simulink model "mavsim_chap10"  (R2018b)
settings: Solver=ode15s  StartTime=0.0  StopTime=400  RelTol=1e-3  EnableMultiTasking=on
InitFcn:
  | clearvars
  | path(pathdef)
  | addpath('../chap2_animation')
  | addpath('../parameters/')
  | aerosonde_parameters
  | simulation_parameters
  | wind_parameters
  | sensor_parameters
  | ekf_parameters
  | addpath('../chap3_kinematics')
  | addpath('../chap4_forces')
  | addpath('../chap5_linear')
  | addpath('../chap6_autopilot')
  | compute_autopilot_gains
  | addpath('../chap7_sensors')
  | addpath('../chap8_estimation')
  | addpath('../chap10_follower')
undefined symbols (not defined in the file or in its folder): AP, autopilot, drawPathError, EKF, estimate_states, forces_moments, MAV, path_follow, path_manager_chap10, SENSOR, SIM, true_states, WIND
libraries: simulink x3
settings Model: Creator=beard  LastModifiedBy=Brandon
settings DataIOCC: LimitDataPoints=on  SaveFormat=Array  SignalLoggingSaveFormat=ModelDataLogs
settings OptimizationCC: ExpressionDepthLimit=2147483647  InitFltsAndDblsToZero=on  LifeSpan=inf
settings DebuggingCC: UnderspecifiedInitializationDetection=Classic  MergeDetectMultiDrivingBlocksExec=none  SolverPrmCheckMsg=warning  FcnCallInpInsideContextMsg=warning  AllowSymbolicDim=off  StateNameClashWarn=warning  SFUnexpectedBacktrackingDiag=warning  SFNoUnconditionalDefaultTransitionDiag=warning  SFExecutionAtInitializationDiag=none
settings HardwareCC: ProdBitPerPointer=32  ProdBitPerSizeT=32  ProdBitPerPtrDiffT=32  ProdLargestAtomicFloat=None  ProdIntDivRoundTo=Undefined  ProdEndianess=Unspecified  ProdWordSize=32  ProdHWDeviceType=32-bit Generic
settings ModelReferenceCC: PropagateSignalLabelsOutOfModel=off
settings SFSimCC: SimUseLocalCustomCode=off  SimParseCustomCode=off
settings RTWCC: RTWUseLocalCustomCode=off
settings CodeAppCC: StateflowObjectComments=on
settings GRTTargetCC: TargetLangStandard=C89/C90 (ANSI)  GeneratePreprocessorConditionals=Disable all  CombineOutputUpdateFcns=off  GRTInterface=on
settings ConfigComp: CovMetricSettings=dw  CovHtmlReporting=on  CovSaveCumulativeToWorkspaceVar=on  CovSaveSingleToWorkspaceVar=on  CovExternalEMLEnable=off  CovSFcnEnable=off

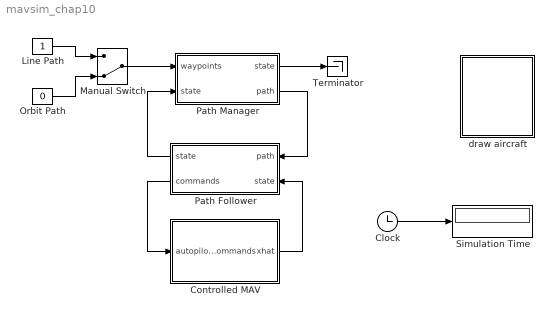
== system mavsim_chap10 ==
  Clock : Clock
  Controlled MAV : Subsystem
      mask Display: image(imread('batcam.png'))
  Line Path : Constant
      settings: AttributesFormatString=%<Name>
  Manual Switch : ManualSwitch  CurrentSetting=0
  Orbit Path : Constant  Value=0
      settings: AttributesFormatString=%<Name>
  Path Follower : Subsystem
  Path Manager : Subsystem
  Simulation Time : Display
  Terminator : Terminator
  draw aircraft : Subsystem
      mask Display: image(imread('tv.jpg'))
  wires:
  Clock/1 -> Simulation Time/1
  Path Manager/2(path) -> Path Follower/1(path)
  Path Follower/2(commands) -> Controlled MAV/1(autopilot commands)
  Controlled MAV/1(xhat) -> Path Follower/2(state)
  Path Follower/1("state ") -> Path Manager/2(state)
  Path Manager/1("state ") -> Terminator/1
  Line Path/1 -> Manual Switch/1
  Orbit Path/1 -> Manual Switch/2
  Manual Switch/1 -> Path Manager/1(waypoints)

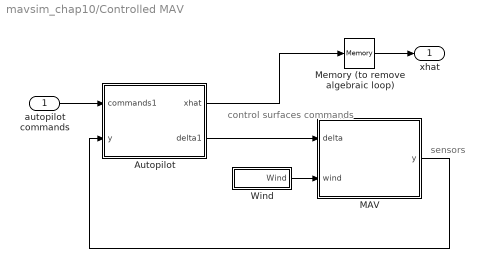
== system mavsim_chap10/Controlled MAV ==
  note: sensors
  note: control surfaces
      | commands
  autopilot commands : Inport
  Autopilot : Subsystem
      mask Display: image(imread('kestrel.jpg'))
  MAV : Subsystem
      mask Display: image(imread('batcam.png'))
  Memory (to remove algebraic loop) : Memory
  Wind : Subsystem
  xhat : Outport
  wires:
  Wind/1(Wind) -> MAV/2(wind)
  MAV/1(y) -> Autopilot/2(y)
  autopilot commands/1 -> Autopilot/1(commands1)
  Memory (to remove algebraic loop)/1 -> xhat/1
  Autopilot/2(delta1) -> MAV/1(delta)
  Autopilot/1(xhat) -> Memory (to remove algebraic loop)/1

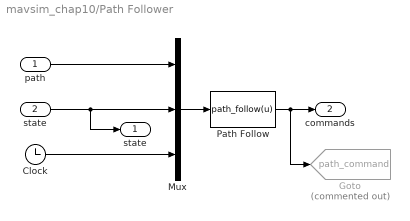
== system mavsim_chap10/Path Follower ==
  path : Inport
  state : Inport  Port=2
  Clock : Clock
  Goto : Goto  Commented=on  GotoTag=path_command  TagVisibility=global
  Mux : Mux  Inputs=3
  Path Follow : MATLABFcn  MATLABFcn=path_follow(u)  OutputDimensions=4  SampleTime=SIM.ts_control
  "state " : Outport
  commands : Outport  Port=2
  wires:
  Path Follow/1 -> commands/1, Goto/1
  Mux/1 -> Path Follow/1
  path/1 -> Mux/1
  Clock/1 -> Mux/3
  state/1 -> Mux/2, "state "/1

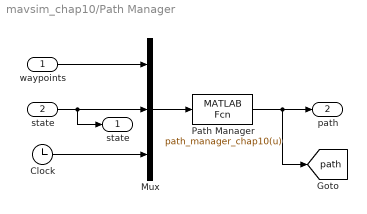
== system mavsim_chap10/Path Manager ==
  waypoints : Inport
  state : Inport  Port=2
  Clock : Clock
  Mux : Mux  Inputs=3
  Path Manager : MATLABFcn  MATLABFcn=path_manager_chap10(u)  OutputDimensions=13  SampleTime=SIM.ts_control
  "state " : Outport
  path : Outport  Port=2
  tag scope: path=global
  wires:
  Path Manager/1 -> path/1, [path]
  Mux/1 -> Path Manager/1
  Clock/1 -> Mux/3
  state/1 -> Mux/2, "state "/1
  waypoints/1 -> Mux/1

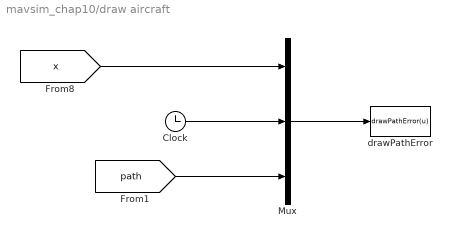
== system mavsim_chap10/draw aircraft ==
  Clock : Clock
  Mux : Mux  Inputs=3
  drawPathError : MATLABFcn  MATLABFcn=drawPathError(u)  OutputDimensions=0  SampleTime=0.1
  wires:
  Clock/1 -> Mux/2
  [x] -> Mux/1
  Mux/1 -> drawPathError/1
  [path] -> Mux/3

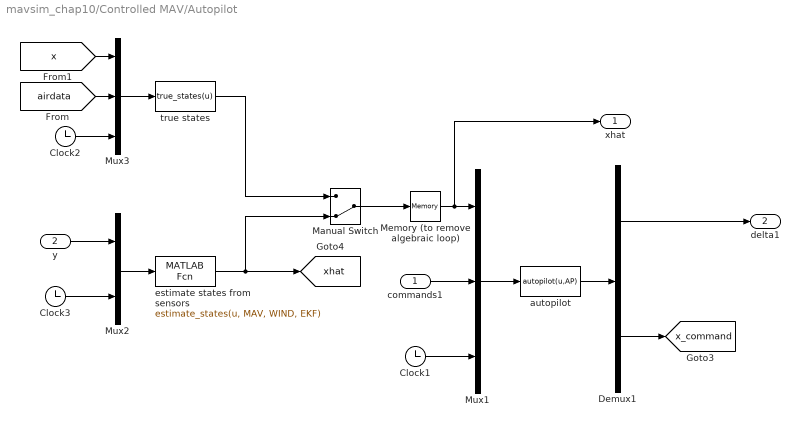
== system mavsim_chap10/Controlled MAV/Autopilot ==
  commands1 : Inport
  y : Inport  Port=2
  Clock1 : Clock
  Clock2 : Clock
  Clock3 : Clock
  Demux1 : Demux  Outputs=[4;12]
  Manual Switch : ManualSwitch  CurrentSetting=0
  Memory (to remove algebraic loop) : Memory
  Mux1 : Mux  Inputs=3
  Mux2 : Mux  Inputs=2
  Mux3 : Mux  Inputs=3
  autopilot : MATLABFcn  MATLABFcn=autopilot(u,AP)  OutputDimensions=4+12  SampleTime=SIM.ts_control
  estimate states from sensors : MATLABFcn  MATLABFcn=estimate_states(u, MAV, WIND, EKF)  OutputDimensions=19  SampleTime=SIM.ts_control
  true states : MATLABFcn  MATLABFcn=true_states(u)  OutputDimensions=19  SampleTime=SIM.ts_simulation
  xhat : Outport
  delta1 : Outport  Port=2
  tag scope: x_command=global, xhat=global
  wires:
  Demux1/1 -> delta1/1
  estimate states from sensors/1 -> [xhat], Manual Switch/2
  Clock3/1 -> Mux2/2
  Clock2/1 -> Mux3/3
  Clock1/1 -> Mux1/3
  [x] -> Mux3/1
  [airdata] -> Mux3/2
  Mux3/1 -> true states/1
  true states/1 -> Manual Switch/1
  Manual Switch/1 -> Memory (to remove algebraic loop)/1
  Memory (to remove algebraic loop)/1 -> xhat/1, Mux1/1
  y/1 -> Mux2/1
  Mux2/1 -> estimate states from sensors/1
  commands1/1 -> Mux1/2
  Demux1/2 -> [x_command]
  autopilot/1 -> Demux1/1
  Mux1/1 -> autopilot/1

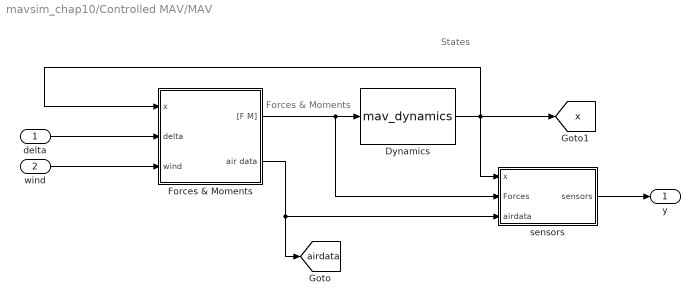
== system mavsim_chap10/Controlled MAV/MAV ==
  note: Forces & Moments
  note: States
  delta : Inport
  wind : Inport  Port=2
  Dynamics : S-Function  FunctionName=mav_dynamics  Parameters=MAV  SFunctionDeploymentMode=off  EnableBusSupport=off
  Forces & Moments : Subsystem
  sensors : Subsystem
  y : Outport
  tag scope: airdata=global, x=global
  wires:
  sensors/1(sensors) -> y/1
  Dynamics/1 -> Forces & Moments/1(x), [x], sensors/1(x)
  Forces & Moments/1("[F M]") -> Dynamics/1, sensors/2(Forces)
  Forces & Moments/2(air data) -> [airdata], sensors/3(airdata)
  delta/1 -> Forces & Moments/2(delta)
  wind/1 -> Forces & Moments/3(wind)

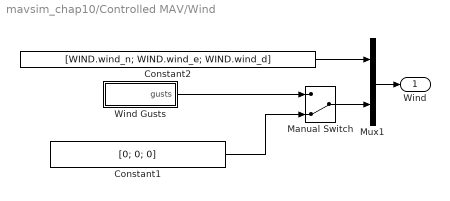
== system mavsim_chap10/Controlled MAV/Wind ==
  Constant1 : Constant  Value=[0; 0; 0]
  Constant2 : Constant  Value=[WIND.wind_n; WIND.wind_e; WIND.wind_d]
  Manual Switch : ManualSwitch  CurrentSetting=0
  Mux1 : Mux  Inputs=2
  Wind Gusts : Subsystem
  Wind : Outport
  wires:
  Mux1/1 -> Wind/1
  Constant2/1 -> Mux1/1
  Constant1/1 -> Manual Switch/2
  Wind Gusts/1(gusts) -> Manual Switch/1
  Manual Switch/1 -> Mux1/2

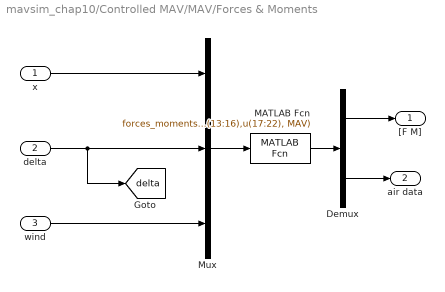
== system mavsim_chap10/Controlled MAV/MAV/Forces & Moments ==
  x : Inport
  delta : Inport  Port=2
  wind : Inport  Port=3
  Demux : Demux  Outputs=[6;6]
  MATLAB Fcn : MATLABFcn  MATLABFcn=forces_moments(u(1:12),u(13:16),u(17:22), MAV)  OutputDimensions=12
  Mux : Mux  Inputs=3
  "[F M]" : Outport
  air data : Outport  Port=2
  tag scope: delta=global
  wires:
  x/1 -> Mux/1
  delta/1 -> [delta], Mux/2
  wind/1 -> Mux/3
  MATLAB Fcn/1 -> Demux/1
  Demux/1 -> "[F M]"/1
  Mux/1 -> MATLAB Fcn/1
  Demux/2 -> air data/1

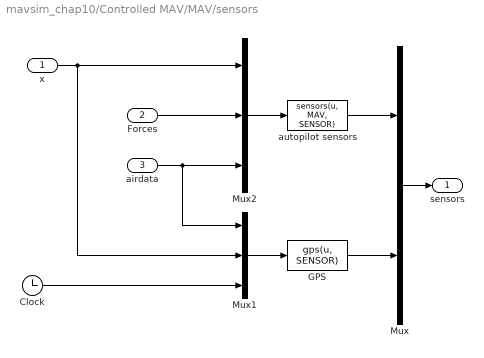
== system mavsim_chap10/Controlled MAV/MAV/sensors ==
  x : Inport
  Forces : Inport  Port=2
  airdata : Inport  Port=3
  Clock : Clock
  GPS : MATLABFcn  MATLABFcn=gps(u, SENSOR)  OutputDimensions=5  SampleTime=SENSOR.ts_gps
  Mux : Mux  Inputs=2
  Mux1 : Mux  Inputs=3
  Mux2 : Mux  Inputs=3
  autopilot sensors : MATLABFcn  MATLABFcn=sensors(u, MAV, SENSOR)  OutputDimensions=8  SampleTime=SIM.ts_simulation
  sensors : Outport
  wires:
  autopilot sensors/1 -> Mux/1
  GPS/1 -> Mux/2
  Mux1/1 -> GPS/1
  Clock/1 -> Mux1/3
  Mux2/1 -> autopilot sensors/1
  Forces/1 -> Mux2/2
  airdata/1 -> Mux2/3, Mux1/1
  Mux/1 -> sensors/1
  x/1 -> Mux2/1, Mux1/2

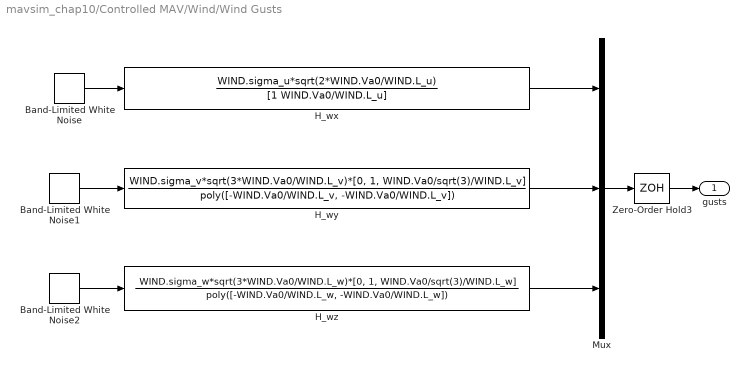
== system mavsim_chap10/Controlled MAV/Wind/Wind Gusts ==
  Band-Limited White Noise : simulink/Sources/Band-Limited White Noise  Cov=[1]  Ts=SIM.ts_simulation  seed=[23341]
  Band-Limited White Noise1 : simulink/Sources/Band-Limited White Noise  Cov=[1]  Ts=SIM.ts_simulation  seed=[23341]
  Band-Limited White Noise2 : simulink/Sources/Band-Limited White Noise  Cov=[1]  Ts=SIM.ts_simulation  seed=[23341]
  H_wx : TransferFcn  Numerator=WIND.sigma_u*sqrt(2*WIND.Va0/WIND.L_u)  Denominator=[1 WIND.Va0/WIND.L_u]
  H_wy : TransferFcn  Numerator=WIND.sigma_v*sqrt(3*WIND.Va0/WIND.L_v)*[0, 1, WIND.Va0/sqrt(3)/WIND.L_v]  Denominator=poly([-WIND.Va0/WIND.L_v, -WIND.Va0/WIND.L_v])
  H_wz : TransferFcn  Numerator=WIND.sigma_w*sqrt(3*WIND.Va0/WIND.L_w)*[0, 1, WIND.Va0/sqrt(3)/WIND.L_w]  Denominator=poly([-WIND.Va0/WIND.L_w, -WIND.Va0/WIND.L_w])
  Mux : Mux  Inputs=3
  Zero-Order Hold3 : ZeroOrderHold  SampleTime=SIM.ts_simulation
  gusts : Outport
  wires:
  Zero-Order Hold3/1 -> gusts/1
  Mux/1 -> Zero-Order Hold3/1
  Band-Limited White Noise2/1 -> H_wz/1
  H_wz/1 -> Mux/3
  Band-Limited White Noise1/1 -> H_wy/1
  H_wy/1 -> Mux/2
  Band-Limited White Noise/1 -> H_wx/1
  H_wx/1 -> Mux/1
